simulink model "ej2"  (Simulink 7.0)
settings: Solver=ode45  StartTime=0.0  StopTime=50.0  RelTol=1e-4
settings Model: Creator=alumno  LastModifiedBy=alumno
settings DataIOCC: Refine=10

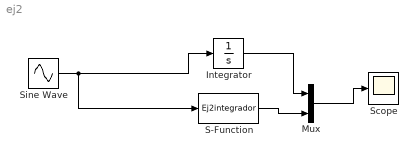
== system ej2 ==
  Integrator : Integrator  InitialCondition=-7  LimitOutput=on  UpperSaturationLimit=5
  Mux : Mux  Inputs=2
  S-Function : S-Function  FunctionName=Ej2integrador  Parameters=-7 5 -10
  Scope : Scope
  Sine Wave : Sin  Amplitude=7  SampleTime=0
  wires:
  S-Function/1 -> Mux/2
  Mux/1 -> Scope/1
  Sine Wave/1 -> S-Function/1, Integrator/1
  Integrator/1 -> Mux/1
